simulink model "jsbsimgui_test"  (Simulink 7.5)
settings: Solver=FixedStepDiscrete  StartTime=0.0  StopTime=15  FixedStep=simulink_delta_t  RelTol=1e-3
values from neighbouring files (symbols this model uses):
  init_aileron = 0    [JSBSim_model_data.m]    (also in model_data.mat)
  init_elevator = 0    [JSBSim_model_data.m]    (also in model_data.mat)
  init_flaps = 0    [JSBSim_model_data.m]    (also in model_data.mat)
  init_gear = 0    [JSBSim_model_data.m]    (also in model_data.mat)
  init_mixture = 0    [JSBSim_model_data.m]    (also in model_data.mat)
  init_rudder = 0    [JSBSim_model_data.m]    (also in model_data.mat)
  init_run_set = 0    [JSBSim_model_data.m]    (also in model_data.mat)
  init_throttle = 0    [JSBSim_model_data.m]    (also in model_data.mat)
undefined symbols (not defined in the file or in its folder): ft, s
libraries: aerolibconvert2 x1
settings Model: Creator=Bri  LastModifiedBy=biffbutkus
settings DataIOCC: SaveOutput=off
settings DebuggingCC: StrictBusMsg=Warning

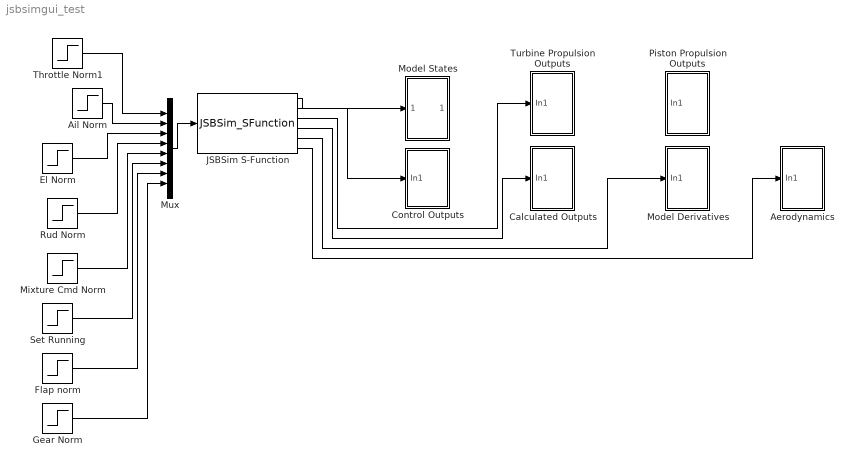
== system jsbsimgui_test ==
  Aerodynamics : Subsystem
  Ail Norm : Step  Time=3  Before=init_aileron  After=init_aileron  SampleTime=0
  Calculated Outputs : Subsystem
  Control Outputs : Subsystem
  El Norm : Step  Time=5  Before=init_elevator  After=init_elevator  SampleTime=0
  Flap norm : Step  Time=0  Before=init_flaps  After=init_flaps  SampleTime=0
  Gear Norm : Step  Time=0  Before=init_gear  After=init_gear  SampleTime=0
  JSBSim S-Function : S-Function  FunctionName=JSBSim_SFunction  Parameters=ac_name, IC_states, IC_controls, IC_delta_t, IC_verbosity,IC_sim_multiplier,IC_solver,IC_fv_sim,IC_fv_trim  EnableBusSupport=off  mask{ac_name='f16', IC_states=[ 925.0006 0.00012509 9.7404 -2.5517e-019 3.056e-019 -2.0001e-020 29999.9998 0.79044 -2.1268 0.00015342 0.01053 -0.003374 ], IC_controls=[ 0.5926 -6.424e-007 -0.071085 5.5102e-007 0.7 1 0 0 ], IC_delta_t=0.00833, IC_verbosity='silent', IC_sim_multiplier=1, IC_solver=[ 3 2 3 2 ], IC_fv_sim=0, IC_fv_trim=0}
      mask prompts: ac_name "AC:"; IC_states "States:"; IC_controls "Controls:"; IC_delta_t "Delta:"; IC_verbosity "Verbosity:"; IC_sim_multiplier "JSBSim Multiplier:"; IC_solver "JSBSim Solvers:"; IC_fv_sim "FlightViz Sim"; IC_fv_trim "FlightViz Trim"
  Mixture Cmd Norm : Step  Time=.1  Before=init_mixture  After=init_mixture  SampleTime=0
  Model Derivatives : Subsystem
  Model States : Subsystem
  Mux : Mux  Inputs=8
  Piston Propulsion Outputs : Subsystem
  Rud Norm : Step  Before=init_rudder  After=init_rudder  SampleTime=0
  Set Running : Step  Time=0  Before=init_run_set  After=init_run_set  SampleTime=0
  Throttle Norm1 : Step  Time=0  Before=init_throttle  After=init_throttle  SampleTime=0
  Turbine Propulsion Outputs : Subsystem
  wires:
  Mux/1 -> JSBSim S-Function/1
  Throttle Norm1/1 -> Mux/1
  El Norm/1 -> Mux/3
  Rud Norm/1 -> Mux/4
  Mixture Cmd Norm/1 -> Mux/5
  Set Running/1 -> Mux/6
  Flap norm/1 -> Mux/7
  Gear Norm/1 -> Mux/8
  Ail Norm/1 -> Mux/2
  JSBSim S-Function/1 -> Model States/1(In1)
  JSBSim S-Function/2 -> Control Outputs/1(In1)
  JSBSim S-Function/3 -> Turbine Propulsion Outputs/1(In1)
  JSBSim S-Function/4 -> Calculated Outputs/1(In1)
  JSBSim S-Function/5 -> Model Derivatives/1(In1)
  JSBSim S-Function/6 -> Aerodynamics/1(In1)

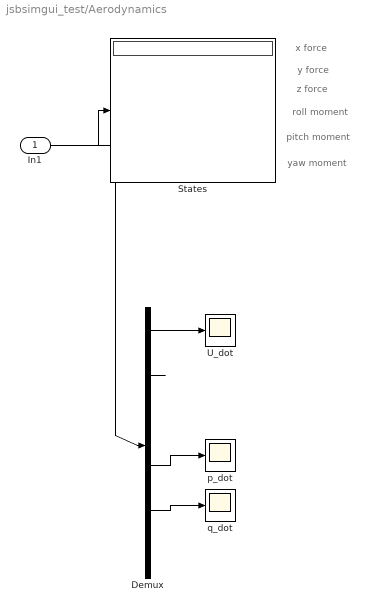
== system jsbsimgui_test/Aerodynamics ==
  note: x force
  note: y force
  note: z force
  note: roll moment
  note: pitch moment
  note: yaw moment
  In1 : Inport
  Demux : Demux  Outputs=6
  States : Display
  U_dot : Scope
  p_dot : Scope
  q_dot : Scope
      settings: SaveName=ScopeData2
  wires:
  In1/1 -> States/1, Demux/1
  Demux/1 -> U_dot/1
  Demux/2 -> ?
  Demux/4 -> p_dot/1
  Demux/5 -> q_dot/1

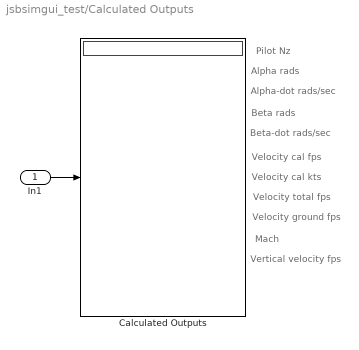
== system jsbsimgui_test/Calculated Outputs ==
  note: Pilot Nz
  note: Alpha rads
  note: Alpha-dot rads/sec
  note: Beta rads
  note: Beta-dot rads/sec
  note: Velocity cal fps
  note: Velocity cal kts
  note: Velocity total fps
  note: Velocity ground fps
  note: Mach
  note: Vertical velocity fps
  In1 : Inport
  Calculated Outputs : Display
  wires:
  In1/1 -> Calculated Outputs/1

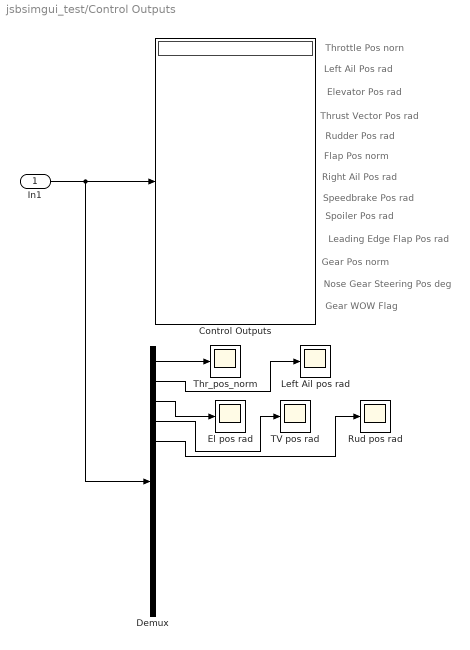
== system jsbsimgui_test/Control Outputs ==
  note: Throttle Pos norn
  note: Left Ail Pos rad
  note: Elevator Pos rad
  note: Rudder Pos rad
  note: Thrust Vector Pos rad
  note: Flap Pos norm
  note: Right Ail Pos rad
  note: Speedbrake Pos rad
  note: Spoiler Pos rad
  note: Leading Edge Flap Pos rad
  note: Gear Pos norm
  note: Nose Gear Steering Pos deg
  note: Gear WOW Flag
  In1 : Inport
  Control Outputs : Display
  Demux : Demux  Outputs=13
  El pos rad : Scope
      settings: SaveName=ScopeData10
  Left Ail pos rad : Scope
      settings: SaveName=ScopeData8
  Rud pos rad : Scope
      settings: SaveName=ScopeData9
  TV pos rad : Scope
      settings: SaveName=ScopeData6
  Thr_pos_norm : Scope
      settings: SaveName=ScopeData7
  wires:
  In1/1 -> Control Outputs/1, Demux/1
  Demux/1 -> Thr_pos_norm/1
  Demux/2 -> Left Ail pos rad/1
  Demux/3 -> El pos rad/1
  Demux/4 -> TV pos rad/1
  Demux/5 -> Rud pos rad/1

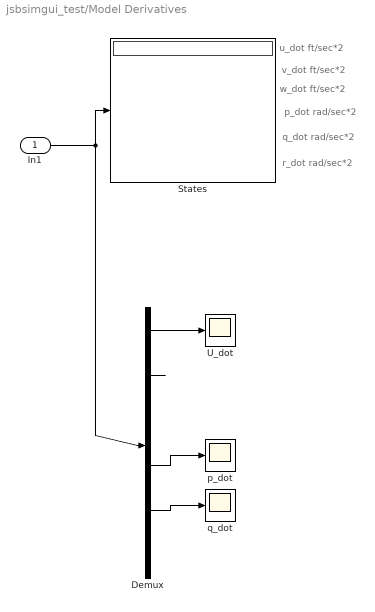
== system jsbsimgui_test/Model Derivatives ==
  note: u_dot ft/sec*2
  note: v_dot ft/sec*2
  note: w_dot ft/sec*2
  note: p_dot rad/sec*2
  note: q_dot rad/sec*2
  note: r_dot rad/sec*2
  In1 : Inport
  Demux : Demux  Outputs=6
  States : Display
  U_dot : Scope
  p_dot : Scope
  q_dot : Scope
      settings: SaveName=ScopeData2
  wires:
  In1/1 -> States/1, Demux/1
  Demux/1 -> U_dot/1
  Demux/2 -> ?
  Demux/4 -> p_dot/1
  Demux/5 -> q_dot/1

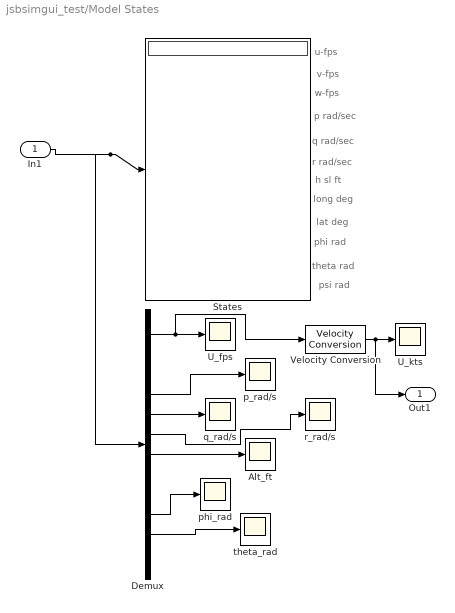
== system jsbsimgui_test/Model States ==
  note: u-fps
  note: v-fps
  note: w-fps
  note: p rad/sec
  note: q rad/sec
  note: r rad/sec
  note: h sl ft
  note: long deg
  note: lat deg
  note: phi rad
  note: theta rad
  note: psi rad
  In1 : Inport
  Alt_ft : Scope
      settings: SaveName=ScopeData3
  Demux : Demux  Outputs=12
  States : Display
  U_fps : Scope
  U_kts : Scope
      settings: SaveName=ScopeData11
  Velocity Conversion : aerolibconvert2/Velocity Conversion  SystemSampleTime=-1  IU=ft/s  OU=kts
  p_rad/s : Scope
  phi_rad : Scope
      settings: SaveName=ScopeData5
  q_rad/s : Scope
      settings: SaveName=ScopeData2
  r_rad/s : Scope
      settings: SaveName=ScopeData12
  theta_rad : Scope
      settings: SaveName=ScopeData4
  Out1 : Outport  OutDataType=fixdt(1, 16)  OutScaling=2^0
  wires:
  In1/1 -> States/1, Demux/1
  Demux/1 -> U_fps/1, Velocity Conversion/1
  Demux/4 -> p_rad/s/1
  Demux/5 -> q_rad/s/1
  Demux/7 -> Alt_ft/1
  Demux/11 -> theta_rad/1
  Demux/10 -> phi_rad/1
  Velocity Conversion/1 -> U_kts/1, Out1/1
  Demux/6 -> r_rad/s/1

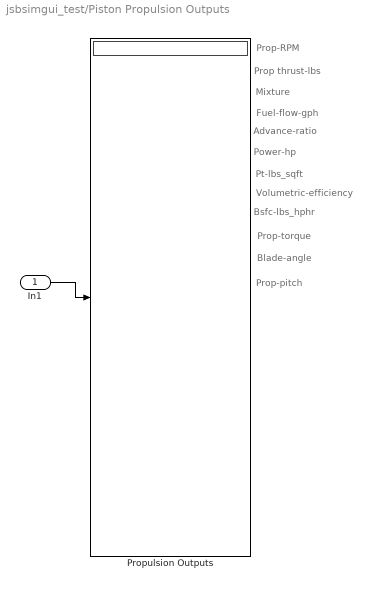
== system jsbsimgui_test/Piston Propulsion Outputs ==
  note: Prop-RPM
  note: Prop thrust-lbs
  note: Mixture
  note: Fuel-flow-gph
  note: Advance-ratio
  note: Power-hp
  note: Pt-lbs_sqft
  note: Bsfc-lbs_hphr
  note: Volumetric-efficiency
  note: Prop-torque
  note: Blade-angle
  note: Prop-pitch
  In1 : Inport
  Propulsion Outputs : Display
  wires:
  In1/1 -> Propulsion Outputs/1

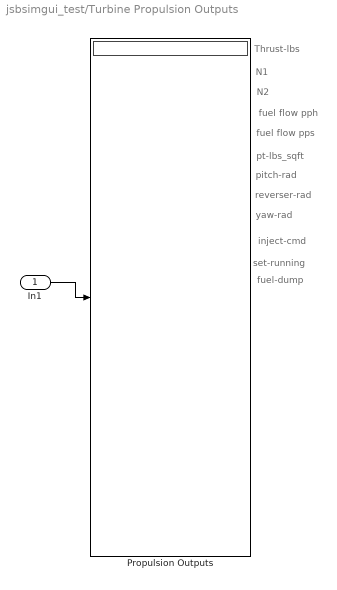
== system jsbsimgui_test/Turbine Propulsion Outputs ==
  note: Thrust-lbs
  note: N1
  note: N2
  note: fuel flow pph
  note: fuel flow pps
  note: pt-lbs_sqft
  note: pitch-rad
  note: reverser-rad
  note: yaw-rad
  note: inject-cmd
  note: set-running
  note: fuel-dump
  In1 : Inport
  Propulsion Outputs : Display
  wires:
  In1/1 -> Propulsion Outputs/1
